simulink library "lib_Convection_MixedBLFlatPlate"  (R2015a)
settings: Solver=ode45  StartTime=0.0  StopTime=10.0  RelTol=1e-3
libraries: simulink x4
settings Model: Creator=jlkratz  LastModifiedBy=jlkratz

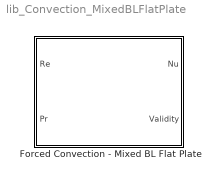
== system lib_Convection_MixedBLFlatPlate ==
  Forced Convection - Mixed BL Flat Plate : Subsystem  mask(TSAT: Mixed BL Flat Plate){Recr_M=500000, IsothermOrIsoflux_M=Isothermal Plate}
      mask prompts: Recr_M "Recr_M - Transition Reynolds Number"
      mask help:
      | This block estimates the average Nusselt number of a mixed boundary layer external flow over an isothermal or isoflux flat plate. The result is for 1 side of the plate. Note that all fluid properrties should be evaluated at film temperature (average of the bulk fluid and surface temperatures). The validity of the result is subject to the following constraints:
      |
      | Re,cr <= Re <= 10^8
      | 0.6 <= Pr <= 60
      |
      | Note that Re,cr is the critical Reynolds number in which the flow transitions to turbulent. The "Validity" output will be 1 if any of the above constraints are not satified and will be 0 otherwise. See the block help menu for additional information.
      mask Help: web(which('Convection_TSAT_MixedBLFlatPlate.html'),'-helpbrowser')
      mask TypeOptions IsothermOrIsoflux_M: Isothermal Plate | Isoflux Plate

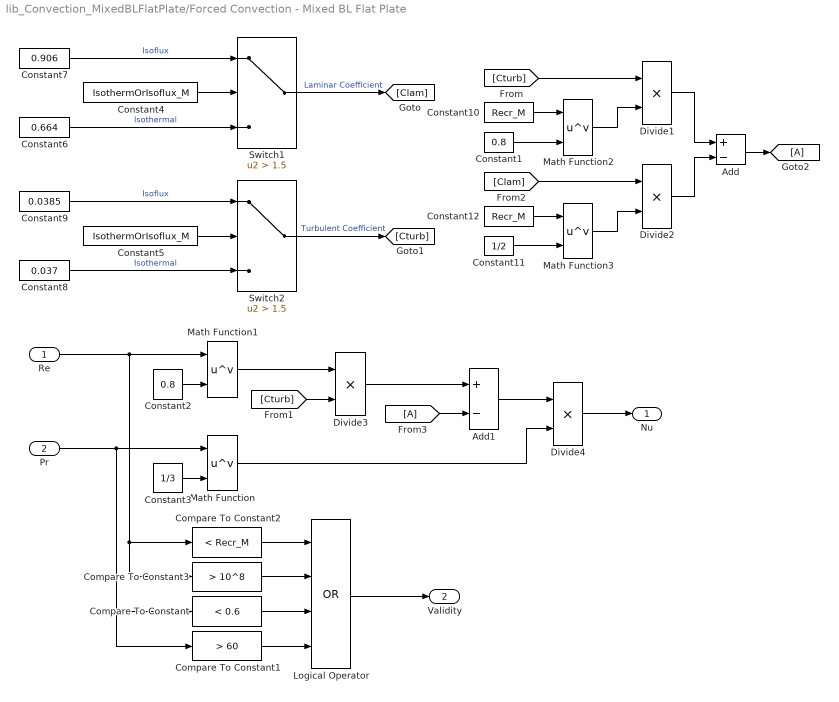
== system lib_Convection_MixedBLFlatPlate/Forced Convection - Mixed BL Flat Plate ==
  Re : Inport
  Pr : Inport  Port=2
  Add : Sum  Inputs=+-
  Add1 : Sum  Inputs=+-
  Compare To Constant : simulink/Logic and Bit Operations/Compare To Constant  relop=<  const=0.6  OutDataTypeStr=boolean
  Compare To Constant1 : simulink/Logic and Bit Operations/Compare To Constant  relop=>  const=60  OutDataTypeStr=boolean
  Compare To Constant2 : simulink/Logic and Bit Operations/Compare To Constant  relop=<  const=Recr_M  OutDataTypeStr=boolean
  Compare To Constant3 : simulink/Logic and Bit Operations/Compare To Constant  relop=>  const=10^8  OutDataTypeStr=boolean
  Constant1 : Constant  Value=0.8
  Constant10 : Constant  Value=Recr_M
  Constant11 : Constant  Value=1/2
  Constant12 : Constant  Value=Recr_M
  Constant2 : Constant  Value=0.8
  Constant3 : Constant  Value=1/3
  Constant4 : Constant  Value=IsothermOrIsoflux_M
  Constant5 : Constant  Value=IsothermOrIsoflux_M
  Constant6 : Constant  Value=0.664
  Constant7 : Constant  Value=0.906
  Constant8 : Constant  Value=0.037
  Constant9 : Constant  Value=0.0385
  Divide{1..4} (4 alike) : Product  Inputs=**
  Logical Operator : Logic  Operator=OR  Inputs=4  AllPortsSameDT=off  OutDataTypeStr=boolean
  Math Function{,1..3} (4 alike) : Math  Operator=pow  SaturateOnIntegerOverflow=on
  Switch1 : Switch  Criteria=u2 > Threshold  Threshold=1.5
  Switch2 : Switch  Criteria=u2 > Threshold  Threshold=1.5
  Nu : Outport
  Validity : Outport  Port=2
  wires:
  Divide4/1 -> Nu/1
  Math Function/1 -> Divide4/2
  Add1/1 -> Divide4/1
  [A] -> Add1/2
  Divide3/1 -> Add1/1
  Math Function1/1 -> Divide3/1
  [Cturb] -> Divide3/2
  Add/1 -> [A]
  Divide2/1 -> Add/2
  Divide1/1 -> Add/1
  Constant12/1 -> Math Function3/1
  Math Function3/1 -> Divide2/2
  [Clam] -> Divide2/1
  Constant11/1 -> Math Function3/2
  Constant10/1 -> Math Function2/1
  Math Function2/1 -> Divide1/2
  [Cturb] -> Divide1/1
  Constant1/1 -> Math Function2/2
  Switch2/1 -> [Cturb]  "Turbulent Coefficient"
  Switch1/1 -> [Clam]  "Laminar Coefficient"
  Constant9/1 -> Switch2/1  "Isoflux"
  Constant8/1 -> Switch2/3  "Isothermal"
  Constant5/1 -> Switch2/2
  Constant6/1 -> Switch1/3  "Isothermal"
  Constant7/1 -> Switch1/1  "Isoflux"
  Constant4/1 -> Switch1/2
  Logical Operator/1 -> Validity/1
  Compare To Constant1/1 -> Logical Operator/4
  Compare To Constant/1 -> Logical Operator/3
  Compare To Constant3/1 -> Logical Operator/2
  Compare To Constant2/1 -> Logical Operator/1
  Constant2/1 -> Math Function1/2
  Constant3/1 -> Math Function/2
  Pr/1 -> Compare To Constant/1, Compare To Constant1/1, Math Function/1
  Re/1 -> Math Function1/1, Compare To Constant3/1, Compare To Constant2/1
